simulink model "simscape_16_nodes_projection"  (R2022b)
settings: Solver=VariableStepAuto  StartTime=0.0  StopTime=0.1  RelTol=1e-3
values from neighbouring files (symbols this model uses):
  fuzhu_ini = x_ini(1:N)    [stepchange_timevarying_change_initial_document.m]
  lambda_ini = zeros(N*(BN+N+1),1)    [stepchange_timevarying_change_initial_document.m]
  Lineindex1 = zeros(BN,2)    [stepchange_timevarying_change_initial_document.m]
  Lineindex2 = zeros(BN,3)    [stepchange_timevarying_change_initial_document.m]
  LoadI = [30.0;15.0;30.0;26.0;         18.9;22.8;29.6;32.1;         22.6;27.6;16.5;19.9;         26.5;19.4;22.7;24.9]    [stepchange_timevarying_change_initial_document.m]
  LoadZ = diag([16.7;50.0;16.7;20.0;              25.0;16.0;14.2;29.4;              18.5;19.6;22.6;25.6;              23.4;26.4;25.2;33.7])    [stepchange_timevarying_change_initial_document.m]
  nu_ini = [-0.00758212493845042	-0.0182492317603708	0.00714905390846842	0.0186908981861182          -0.00758212493845042	-0.0182492317603708	0.00714905390846842	0.0186908981861182          -0.00758212493845042	-0.0182492317603708	0.00714905390846842	0.0186908981861182          -0.00758212493845042	-0.0182492317603708	0.00714905390846842	0.0186908981861182]'    [stepchange_timevarying_change_initial_document.m]
  theta_ini = zeros(N*(BN+N+1),1)    [stepchange_timevarying_change_initial_document.m]
  u_ini = [378.9289  380.4146  379.7396  379.2243  380.1955  381.1042         379.9247  379.8974  380.0252  380.4045  379.6763  379.8341         380.1194  380.5682  379.3881  379.9696]'    [stepchange_timevarying_change_initial_document.m]
  x_hat_ini = [14.515064754915	3.95935897697232	32.9787419273847	14.9071228299889             37.6257931691129	61.1095883901259	41.4721611959256	33.6364102939300             44.9867290171943	52.8132621486412	28.1355733315040	33.0707668633162             36.6024320622732	49.3936276267038	2.38033527987224	36.4476162672594             378.638597580330	380.343321138855	379.211948658584	379.000752058610              ...(+639 chars)    [stepchange_timevarying_change_initial_document.m]
libraries: fl_lib x204, nesl_utility x101, spspowerguiLib x1
(part 3 of 3)

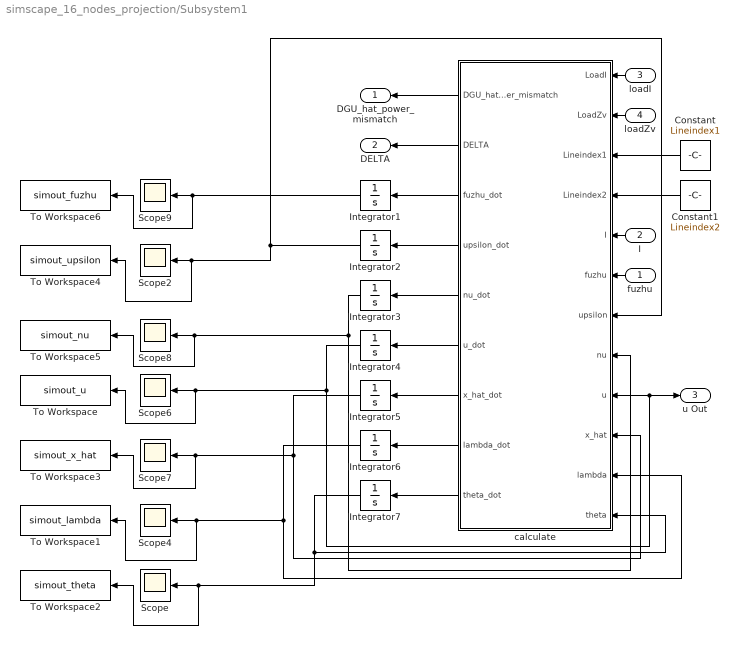
== system simscape_16_nodes_projection/Subsystem1 ==
  fuzhu : Inport
  I : Inport  Port=2
  loadI : Inport  Port=3
  loadZv : Inport  Port=4
  Constant : Constant  Value=Lineindex1
  Constant1 : Constant  Value=Lineindex2
  Integrator1 : Integrator  InitialCondition=fuzhu_ini
  Integrator2 : Integrator  InitialCondition=fuzhu_ini
  Integrator3 : Integrator  InitialCondition=nu_ini
  Integrator4 : Integrator  InitialCondition=u_ini
  Integrator5 : Integrator  InitialCondition=x_hat_ini
  Integrator6 : Integrator  InitialCondition=lambda_ini
  Integrator7 : Integrator  InitialCondition=theta_ini
  Scope{,2,4,6..9} (7 alike) : Scope
  To Workspace : ToWorkspace  VariableName=simout_u  SaveFormat=Timeseries  SampleTime=-1
  To Workspace1 : ToWorkspace  VariableName=simout_lambda  SaveFormat=Timeseries  SampleTime=-1
  To Workspace2 : ToWorkspace  VariableName=simout_theta  SaveFormat=Timeseries  SampleTime=-1
  To Workspace3 : ToWorkspace  VariableName=simout_x_hat  SaveFormat=Timeseries  SampleTime=-1
  To Workspace4 : ToWorkspace  VariableName=simout_upsilon  SaveFormat=Timeseries  SampleTime=-1
  To Workspace5 : ToWorkspace  VariableName=simout_nu  SaveFormat=Timeseries  SampleTime=-1
  To Workspace6 : ToWorkspace  VariableName=simout_fuzhu  SaveFormat=Timeseries  SampleTime=-1
  calculate : MATLAB Function  TreatAsAtomicUnit=on
  DGU_hat_power_mismatch : Outport
  DELTA : Outport  Port=2
  u Out : Outport  Port=3
  wires:
  Integrator3/1 -> To Workspace5/1, Scope8/1, calculate/8(nu)
  Integrator6/1 -> To Workspace1/1, Scope4/1, calculate/11(lambda)
  calculate/9(theta_dot) -> Integrator7/1
  Constant/1 -> calculate/3(Lineindex1)
  calculate/6(u_dot) -> Integrator4/1
  calculate/3(fuzhu_dot) -> Integrator1/1
  Constant1/1 -> calculate/4(Lineindex2)
  Integrator4/1 -> u Out/1, calculate/9(u), To Workspace/1, Scope6/1
  Integrator5/1 -> calculate/10(x_hat), To Workspace3/1, Scope7/1
  fuzhu/1 -> calculate/6(fuzhu)
  calculate/4(upsilon_dot) -> Integrator2/1
  Integrator1/1 -> To Workspace6/1, Scope9/1
  I/1 -> calculate/5(I)
  Integrator2/1 -> To Workspace4/1, Scope2/1, calculate/7(upsilon)
  calculate/8(lambda_dot) -> Integrator6/1
  calculate/5(nu_dot) -> Integrator3/1
  Integrator7/1 -> calculate/12(theta), To Workspace2/1, Scope/1
  calculate/7(x_hat_dot) -> Integrator5/1
  calculate/2(DELTA) -> DELTA/1
  calculate/1(DGU_hat_power_mismatch) -> DGU_hat_power_mismatch/1
  loadI/1 -> calculate/1(LoadI)
  loadZv/1 -> calculate/2(LoadZv)

== matlab function simscape_16_nodes_projection/Subsystem1/calculate ==
  data: LoadI input; LoadZv input; DGU_hat_power_mismatch output; DELTA output; fuzhu_dot output; Lineindex1 input; Lineindex2 input; I input; fuzhu input; upsilon input; nu input; u input; x_hat input; lambda input; theta input; upsilon_dot output; nu_dot output; u_dot output; x_hat_dot output; lambda_dot output; theta_dot output
function [ DGU_hat_power_mismatch,DELTA,fuzhu_dot,upsilon_dot,nu_dot,u_dot,x_hat_dot,lambda_dot,theta_dot] =fcn(LoadI,LoadZv,Lineindex1,Lineindex2, I,fuzhu,upsilon,nu,u,x_hat,lambda,theta)

%======================================Algorithm parameters===================================

kappa=10;

N=16;

epsilon=2; 

varepsilon=50; 

%=========================================Graph parameters====================================

Line1=[1;1;2;2;3;3;4;4; ...
       5;5;6;6;7;7;8;8; ...
       9;9;10;10;11;11;12;12; ...
       13;13;14;14;15;15;16;16; ...
       3;3;8;8;9;9;14;14];

Line2=[2;4;1;3;2;4;1;3; ...
       6;8;5;7;6;8;5;7; ...
       10;12;9;11;10;12;9;11; ...
       14;16;13;15;14;16;13;15; ...
       8;14;3;9;8;14;3;9];

BN=size(Line1,1)/2;

GN=size(Line1,1); 

Adjacent=zeros(N,N);                                                       %adjacent matrix 

for i=1:GN
     
         Adjacent(Line1(i),Line2(i))=1;                                    %adjacent matrix 
         
         Adjacent(Line2(i),Line1(i))=1;                                    %adjacent matrix 
              
end    
    
Degree=diag(Adjacent*ones(N,1));                                           %Degree matrix

Lap=200*(Degree-Adjacent);                                                 %Laplacian matrix

Lap_BN_plus_N=kron(Lap,eye(BN+N+1));                                       %Laplacian matrix kronect

Lap_BN=kron(Lap,eye(BN));                                                  %Laplacian matrix kronect

%-------------------------------------Construct incidence matrix------------------------------ 

% Lineindex1=zeros(BN,2);                                                    %initial matrix
% 
% Lineindex2=zeros(BN,3);
% 
% kk=1;                                                                      %initial count number
% 
% for i=1:GN                                                                 %set line belongs index, i.e. \mathcal{C}_i
% 
%     if isempty(intersect([min(Line1(i),Line2(i)),max(Line1(i),Line2(i))],Lineindex1,'row'))
% 
%         Lineindex1(kk,:)=[min(Line1(i),Line2(i)),max(Line1(i),Line2(i))];     
%         
%         Lineindex2(kk,:)=[Lineindex1(kk,:),kk];                            %include line number
% 
%         kk=kk+1;
% 
%     end
% 
% end

Lineindex=zeros(BN,4);

kk=1;

for j=1:N                                                                 %initial count number
    
    for i=1:BN
        
        if Lineindex1(i,1)==j

            Lineindex(kk,:)=[j,Lineindex2(i,:)];                            %Lines are managed by agent j
            
            kk=kk+1;
            
        end

    end

end

NCLN=zeros(N,1);

for i=1:N                                                                  %How many lines are under control of each agent
    
    if find(Lineindex(:,1)==i)~=0
    
        NCLN(i,1)=size(find(Lineindex(:,1)==i),1);                               %node control's lines number
        
    else
        
         NCLN(i,1)=0;                                                      %No line is under control of this node
        
    end
    
end

B=zeros(N,BN);                                                             %initial incidence matrix

for i=1:BN

    B(Lineindex1(i,1),i)=1;                                                %Set the initial node as 1   
    
    B(Lineindex1(i,2),i)=-1;                                                %Set the end node as -1 
    
end

%=========================================Power network parameters====================================

R=diag([2.0 1.8 1.6 1.5 ...
        2.2 1.9 2.6 2.8 ...
        1.7 1.9 2.4 2.3 ...
        2.6 2.1 2.0 1.9]*10^-2);

L=diag([1.8 2.0 3.0 2.2 ...
        2.2 2.3 1.9 2.5 ...
        1.7 2.2 2.3 2.9 ...
        2.3 2.5 1.9 3.0]*10^-3);

C=diag([2.2 1.9 2.5 1.7 ...
        1.8 2.2 2.9 3.1 ...
        1.7 2.5 2.6 1.9 ...
        1.9 1.9 2.2 2.3]*10^-3);

L_l=diag([2.1 2.0 3.0 2.2 ...
          2.3 2.6 2.0 1.9 ...
          2.3 2.5 2.8 2.4 ...
          2.3 2.5 2.6 2.4 ...
          2.1 2.3 2.5 2.6]*10^-6);

R_l=diag([7 5 8 6 ...
          8 8 5 6 ...
          8 7 6 7 ...
          8 7 8 5 ...
          7 6 7 8]*10^-2);

LoadZ=diag(LoadZv);

% LoadZ=diag([16.7;50;16.7;20]);
% 
% LoadI=[30;15;30;26];

%LoadI=zeros(4,1);

%LoadI=ones(4,1)

Lineconstrants=15*ones(BN,1);                                              %Transmission line limits

Line_loss=300;                                                               %Transmission line power loss limits

V_r=[380.16  381.21  380.08  380.13 ...
     380.16  381.21  380.08  380.13 ...
     380.16  381.21  380.08  380.13 ...
     380.16  381.21  380.08  380.13]';                             %Reference voltage 1    

V_hat_low=(380-3)*ones(N,1);                                                 %Voltage lower bound  

V_hat_up=(380+3)*ones(N,1);                                                  %Voltage upper bound

pr=0.005;                                                                  %Curnot model parameter

l=2.5;                                                                       %Curnot model parameter

r=[1.06 1.03 1.05 1.04 ...
   1.06 1.03 1.05 1.04 ...
   1.06 1.03 1.05 1.04 ...
   1.06 1.03 1.05 1.04];                                  %initial r_i

A_r=kron(diag(r),eye(N+BN+1));                                              %initial kenonect r

alpha_I=[10.6000   10.1000   10.2900   10.5000 ...
         10.7824   10.9083   10.1385   10.8665 ...
         10.6003   10.5795    9.6473   11.3287 ...
         10.3660   10.9800   10.2331   10.5255]'; 
 
alpha_V=[0.7500    0.6200    0.8500    0.9300 ...
         0.7733    1.2066    0.8871    1.2904 ...
         0.3321    0.3491   -0.0031    1.7190 ...
         1.0019    0.5118    1.1699    1.0789]';                            %Optimization model parameter  xxxxxxxxxxxxxxxxxx

alpha_u=[1.1000    1.4000    1.8000    1.1000 ...
         1.1543    1.9921    1.9570    1.2813 ...
         1.3085    1.4853    1.8793    0.6247 ...
         1.8416    2.1018    1.5065    0.9843]';                            %Optimization model parameter  xxxxxxxxxxxxx

alpha_I_l=[1.4000    1.9000    1.7000    1.9000 ...
           0.5764    1.2538    1.6124    1.6703 ...
           0.7906    1.3172    1.8742    1.4831 ...
           0.3893    1.4932    1.7202    1.4751 ...
           1.1780    1.9363    2.0859    1.8746]';                         %Optimization model parameter  xxxxxxxxxx
%=========================================  Microgrid matrix  ===================================

DGU_inverse=blkdiag(L^-1,C^-1,L_l^-1);

M=[-R,-eye(N),zeros(N,BN); eye(N),-LoadZ^-1,B;zeros(BN,N),-B',-R_l];

A=[eye(N),     -LoadZ^-1,   B; zeros(BN,N),  R_l^-1*B',   eye(BN); zeros(1,N),  zeros(1,N),   V_r'*B ];

s_A=zeros(N*(N+BN+1),1);

for i=1:N

    s_A((i-1)*(N+BN+1)+1:i*(N+BN+1))=[zeros(N,1);zeros(BN,1);Line_loss/N];

    s_A((i-1)*(N+BN+1)+i)=LoadI(i);

end

%%=========================================  Loacal constraints  ===================================

F_x_I=zeros(BN,BN);  %xxxxxxxxxxxxxxxxxxxxxxxx

        for i=1:N 

            if NCLN(i,1)~=0

                choose_line=find(Lineindex(:,1)==i);

                for j=1:NCLN(i,1)                                          %The numbers of the controlled line of agent i

                    aa=Lineindex(choose_line(j),4);                                  %choose which line
        
                    F_x_I(aa,aa)=r(i).*alpha_I_l(aa);    
        
                end

            end
            
        end

F_x=blkdiag(diag(r)*diag(alpha_I)+diag(r)*pr*diag(V_r),diag(r)*diag(alpha_V),F_x_I);

%---------------------------------ojection local constraint setting--------------------------------

normal_vector_nonstandar=zeros(3*N,1);

normal_vector=zeros(3*N,1);

reference_vector_low_1=zeros(3*N,1);

reference_vector_low_2=zeros(3*N,1);

bound_vector_low_nonstandar=zeros(3*N,1);

bound_low_vector=zeros(3*N,1);

reference_vector_up_1=zeros(3*N,1);

reference_vector_up_2=zeros(3*N,1);

bound_vector_up_nonstandar=zeros(3*N,1);

bound_up_vector=zeros(3*N,1);


for i=1:N                                                                  % for all nodes calculate the normal vector
    
    normal_vector_nonstandar((i-1)*3+1:i*3)=[-1/R(i,i);1;1/R(i,i)];                    % caulculate the Projection normal vector
    
    normal_vector((i-1)*3+1:i*3)=(1/norm(normal_vector_nonstandar((i-1)*3+1:i*3),2))...            % normalized the Projection normal vector
                     *[-1/R(i,i);1;1/R(i,i)];
    
end    

for i=1:N                                                                               % for all nodes calculate the bound vector
    
    reference_vector_low_1((i-1)*3+1:i*3)=[V_hat_low(i);0;V_hat_low(i)];                            % first reference node located at the lower bound
    
    reference_vector_low_2((i-1)*3+1:i*3)=[0;-V_hat_low(i)/R(i,i);V_hat_low(i)];                    % second reference node located at the lower bound
    
    bound_vector_low_nonstandar((i-1)*3+1:i*3)=reference_vector_low_1((i-1)*3+1:i*3)-reference_vector_low_2((i-1)*3+1:i*3); % vector along the lower bound
    
    bound_low_vector((i-1)*3+1:i*3)=(1/norm(bound_vector_low_nonstandar((i-1)*3+1:i*3),2))...                   % normalized the vector along the lower bound
                         *bound_vector_low_nonstandar((i-1)*3+1:i*3);
                    
    reference_vector_up_1((i-1)*3+1:i*3)=[V_hat_up(i);0;V_hat_up(i)];                               % first reference node located at the upper bound
    
    reference_vector_up_2((i-1)*3+1:i*3)=[0;-V_hat_up(i)/R(i,i);V_hat_up(i)];                       % second reference node located at the upper bound
    
    bound_vector_up_nonstandar((i-1)*3+1:i*3)=reference_vector_up_1((i-1)*3+1:i*3)-reference_vector_up_2((i-1)*3+1:i*3);    % vector along the upper bound
    
    bound_up_vector((i-1)*3+1:i*3)=(1/norm(bound_vector_up_nonstandar((i-1)*3+1:i*3),2))...                     % normalized the vector along the upper bound
                       *bound_vector_up_nonstandar((i-1)*3+1:i*3);
end  


%---------------------------------------dynamic extra calculate--------------------------------------

col_r_i_A_i_top_lambda_i=zeros(2*N+BN,1);

col_Ax_hat_s_A=zeros(N*(N+BN+1),1);

A_i_I_l=zeros(N*(N+BN+1),1);

A_I_l_choose=zeros(BN,1);

        for i=1:N

            A_i_I_l((i-1)*(N+BN+1)+1:i*(N+BN+1))=zeros(N+BN+1,1);

            if NCLN(i,1)~=0

                    check_line_no=find(Lineindex(:,1)==i);

                for j=1:NCLN(i,1)                                          %The numbers of the controlled line of agent i

                    aa=Lineindex(check_line_no(j),4);                                  %choose which line

                    zhong_jian=A_i_I_l((i-1)*(N+BN+1)+1:i*(N+BN+1));
        
                    A_i_I_l((i-1)*(N+BN+1)+1:i*(N+BN+1))=zhong_jian+A(:,2*N+aa)*x_hat(2*N+aa);    %calculate the value of sum B_iI_l_i
                    
                    A_I_l_choose(aa)=r(i)*(A(:,2*N+aa)'*lambda(1+(i-1)*(N+BN+1):i*(N+BN+1)));
        
                end

            end            
            
                col_Ax_hat_s_A(1+(i-1)*(N+BN+1):i*(N+BN+1))=r(i)*(A(:,i)*x_hat(i)+A(:,N+i)*x_hat(i+N)+A_i_I_l((i-1)*(N+BN+1)+1:i*(N+BN+1))-s_A((i-1)*(N+BN+1)+1:i*(N+BN+1)));

                col_r_i_A_i_top_lambda_i(i)=r(i).*A(:,i)'*lambda(1+(i-1)*(N+BN+1):i*(N+BN+1));

                col_r_i_A_i_top_lambda_i(i+N)=r(i).*A(:,N+i)'*lambda(1+(i-1)*(N+BN+1):i*(N+BN+1));

        end

        for i=1:BN

                col_r_i_A_i_top_lambda_i(i+2*N)=A_I_l_choose(i);

        end

%       x_dot=DGU_inverse*M*x+DGU_inverse*[u+0.8*(fuzhu-x(1:N));-LoadI;zeros(BN,1)];                    %Dynamic for microgrid's states

        fuzhu_dot=-100*(fuzhu-I);
        
        upsilon_dot=(varepsilon*(-(eye(N)+Lap)*upsilon-Lap*nu+N*x_hat(1:N)));

        nu_dot=(varepsilon*(Lap*upsilon));

        u_dot=kappa*(-alpha_u.*u-epsilon*(I-x_hat(1:N)));   %xxxxxx gai guo

        x_hat_dot=kappa*(-F_x*x_hat+[diag(r)*diag(V_r)*(l*ones(N,1)-pr*upsilon);diag(r)*alpha_V.*V_r;zeros(BN,1)]-100*col_r_i_A_i_top_lambda_i);

        lambda_dot=kappa*(100*col_Ax_hat_s_A-A_r*Lap_BN_plus_N*A_r*lambda-A_r*Lap_BN_plus_N*theta);

        theta_dot=kappa*(Lap_BN_plus_N*A_r*lambda);

        %---------------------------------projection local constraint cauculation--------------------------------

        projection_judge=zeros(3*N,1);

        projection_vector=zeros(3*N,1);

        for i=1:N                                                                                                       % for all node
            
            projection_judge((i-1)*3+1:3*i)=[u_dot(i);x_hat_dot(i);x_hat_dot(N+i)];

            projection_vector((i-1)*3+1:3*i)=projection_judge((i-1)*3+1:3*i)-projection_judge((i-1)*3+1:3*i)'*normal_vector((i-1)*3+1:3*i)*normal_vector((i-1)*3+1:3*i);
            
            
            if x_hat(N+i)<=V_hat_low(i) && projection_vector(3*i)<0                                                                                 %the projection vector is on the leftside of the feasible set         
                 
                 projection_vector((i-1)*3+1:3*i)=projection_judge((i-1)*3+1:3*i)'*bound_low_vector((i-1)*3+1:3*i)*bound_low_vector((i-1)*3+1:3*i);                           %projection on lower bound
                
             end
             
             if x_hat(N+i)>=V_hat_up(i) && projection_vector(3*i)>0                                                                                     %the projection vector is on the leftside of the feasible set       
                         
                 projection_vector((i-1)*3+1:3*i)=projection_judge((i-1)*3+1:3*i)'*bound_up_vector((i-1)*3+1:3*i)*bound_up_vector((i-1)*3+1:3*i);                                                   %projection on upper bound
                
             end    
             
             u_dot(i)=projection_vector((i-1)*3+1);                                                                     % recover the u_g_d dynamic
        
             x_hat_dot(i)=projection_vector((i-1)*3+2);                                                                     % recover the I_g_d dynamic
        
             x_hat_dot(N+i)=projection_vector((i-1)*3+3);                                                                     % recover the V_g_d dynamic
        
             
        end

        for i=1:BN
        
            if x_hat(2*N+i)>=Lineconstrants(i) &&  x_hat_dot(2*N+i)>0   

                x_hat_dot(2*N+i)=0;

            elseif x_hat(2*N+i)<=-Lineconstrants(i) &&  x_hat_dot(2*N+i)<0

                x_hat_dot(2*N+i)=0;

            end

        end

%---------------------------------projection coupling constraint cauculation--------------------------------


for i=1:N

    if lambda(i*(N+BN+1))<=0 && lambda_dot(i*(N+BN+1))<0

        lambda_dot(i*(N+BN+1))=0;

    end

end



        DGU_hat_power_mismatch=-u+R*x_hat(1:N)+x_hat(N+1:2*N);


       DELTA=DGU_inverse*M*x_hat+DGU_inverse*[u;-LoadI;zeros(BN,1)];
